simulink model "Tuning_L"  (R2023b)
settings: Solver=FixedStepAuto  StartTime=0.0  StopTime=inf  RelTol=1e-3  EnableMultiTasking=on
values from neighbouring files (symbols this model uses):
  alpha = exp(-Tfs/Ts)    [model_approximation.m]
  Ts = 0.005    [attempt.m]    (also in model_approximation.m; tuning.m)
libraries: mbedblockslib x4, eeStairGenerator x1
settings Model: ExtModeTrigDuration=10  Creator=david  LastModifiedBy=david
settings OptimizationCC: EnhancedBackFolding=on  PassReuseOutputArgsAs=Individual arguments  ZeroExternalMemoryAtStartup=off  ZeroInternalMemoryAtStartup=off  MaxStackSize=64  OptimizeBlockOrder=speed  DifferentSizesBufferReuse=on  OptimizationCustomize=off  EfficientTunableParamExpr=on
settings DebuggingCC: ParameterTunabilityLossMsg=error
settings HardwareCC: ProdBitPerPointer=32  ProdBitPerSizeT=32  ProdBitPerPtrDiffT=32  ProdLargestAtomicInteger=Long  ProdLargestAtomicFloat=Double  ProdWordSize=32  ProdLongLongMode=on  ProdHWDeviceType=ARM Compatible->ARM Cortex
settings SFSimCC: MATLABDynamicMemAlloc=off
settings RTWCC: Description=Embedded Coder  SystemTargetFile=ert.tlc  HardwareBoard=STM32 Nucleo F401RE  TemplateMakefile=ert_default_tmf  Toolchain=GNU Tools for ARM Embedded Processors
settings CodeAppCC: ForceParamTrailComments=on  IgnoreCustomStorageClasses=off  OperatorAnnotations=on  SimulinkDataObjDesc=on  SFDataObjDesc=on  InsertBlockDesc=on
settings ERTTargetCC: ExtModeTransport=3  ExtModeStaticAlloc=on  ExtModeStaticAllocSize=2000  ExtModeMexFile=ext_xcp  ExtModeIntrfLevel=Level2 - Open

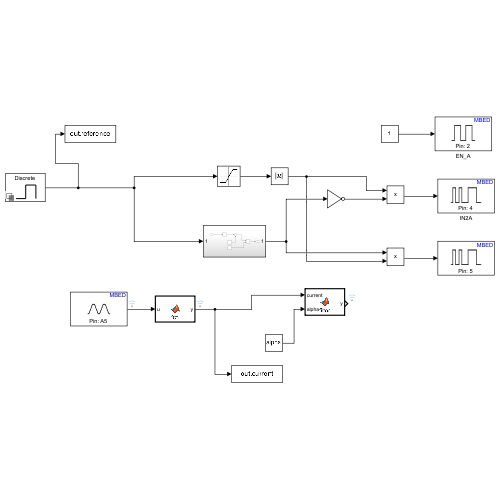
[thumbnail: Simulink's stored preview of the top-level diagram]
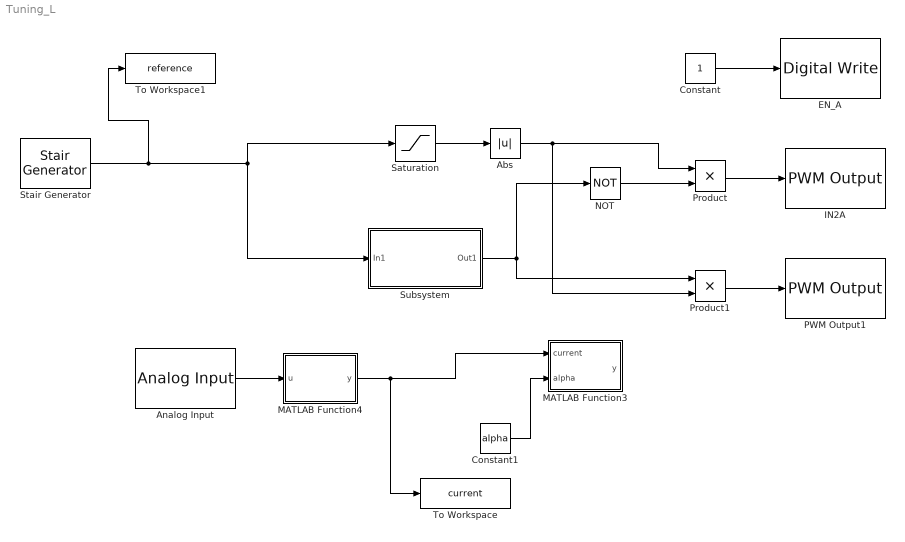
== system Tuning_L ==
  Abs : Abs  SaturateOnIntegerOverflow=off
  Analog Input : mbedblockslib/Analog Input  Pin=A5  ReadResultsOnly=off  ConversionTriggerSource=Software  ExternalTriggerType=uint32( 0 )  OutputDataType=double  EnableConversionCompleteNotify=off  EnableOuputStatus=off  SampleTime=Ts
      settings: LibrarySourceBlock=stmnucleorootlib/Common/Analog Input
  Constant : Constant
  Constant1 : Constant  Value=alpha
  EN_A : mbedblockslib/Digital Write  Pin=2  Direction=output
      settings: LibrarySourceBlock=stmnucleorootlib/Common/Digital Write
  IN2A : mbedblockslib/PWM Output  Pin=4  EnableInputFrequency=off  InitialFrequency=pwmFreq  InitialDutyCycle=50  NotificationType=None
      settings: LibrarySourceBlock=stmnucleorootlib/Common/PWM Output
  MATLAB Function3 : MATLAB Function  TreatAsAtomicUnit=on
  MATLAB Function4 : MATLAB Function  TreatAsAtomicUnit=on
  NOT : Logic  Operator=NOT  IconShape=distinctive  AllPortsSameDT=off  OutDataTypeStr=boolean
  PWM Output1 : mbedblockslib/PWM Output  Pin=5  EnableInputFrequency=off  InitialFrequency=2000  InitialDutyCycle=50  NotificationType=None
      settings: LibrarySourceBlock=stmnucleorootlib/Common/PWM Output
  Product : Product
  Product1 : Product
  Saturation : Saturate  UpperLimit=100  LowerLimit=-100
  Stair Generator : eeStairGenerator/Stair Generator  LabelModeActiveChoice=Discrete  TimeInput=[0 5 10]  AmplitudeInput=[0 100 0]  SampleTime=Ts  RepeatPattern=on  OutDataTypeStr=double
      settings: LibrarySourceBlock=ee_sl_lib/General Control/Stair Generator
  Subsystem : Subsystem
  To Workspace : ToWorkspace  VariableName=current  SaveFormat=Timeseries  SampleTime=-1
  To Workspace1 : ToWorkspace  VariableName=reference  SaveFormat=Timeseries  SampleTime=-1
  wires:
  MATLAB Function4/1(y) -> To Workspace/1, MATLAB Function3/1(current)
  Constant1/1 -> MATLAB Function3/2(alpha)
  Analog Input/1 -> MATLAB Function4/1(u)
  Abs/1 -> Product1/2, Product/1
  Subsystem/1(Out1) -> NOT/1, Product1/1
  Stair Generator/1 -> To Workspace1/1, Subsystem/1(In1), Saturation/1
  NOT/1 -> Product/2
  Product/1 -> IN2A/1
  Product1/1 -> PWM Output1/1
  Saturation/1 -> Abs/1
  Constant/1 -> EN_A/1

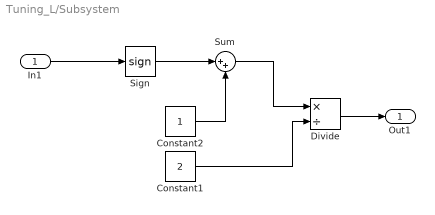
== system Tuning_L/Subsystem ==
  In1 : Inport
  Constant1 : Constant  Value=2
  Constant2 : Constant
  Divide : Product  Inputs=*/
  Sign : Signum
  Sum : Sum  Inputs=|++
  Out1 : Outport
  wires:
  Constant1/1 -> Divide/2
  Sign/1 -> Sum/1
  Constant2/1 -> Sum/2
  In1/1 -> Sign/1
  Sum/1 -> Divide/1
  Divide/1 -> Out1/1

== matlab function Tuning_L/MATLAB Function4 ==
  data: u input; y output
function y = fcn(u)
    v_input = u*3.3;
    current = (1/0.185)*(v_input-2.5);
y = current

== matlab function Tuning_L/MATLAB Function3 ==
  data: current input; y output; alpha input
function y = filter(current, alpha)
    persistent current_old current_filtered_old;

    if isempty(current_old)
        current_old = current;
        current_filtered_old = 0;
    else
        current_temp = current;
        current = alpha*current_filtered_old + (1 - alpha) *current_old;
        current_old = current_temp;
        current_filtered_old = current;
    end

y = current;
